simulink model "ROPOD_Control_SIM"  (R2017b)
settings: Solver=VariableStepAuto  StartTime=0.0  StopTime=inf  RelTol=1e-3
values from neighbouring files (symbols this model uses):
  AgentNumber = 1    [init_model.m]
  FFtheta_intia = 0    [init_model.m]
  FFxy_mass = 0*80    (= 0)    [init_model.m]
  flock_FFtheta_friction = 50    [init_model.m]
  flock_FFxy_friction = 100    [init_model.m]
  I_fhz_ddelta_cntr = 0    [init_model.m]
  I_fhz_dtheta_cntr = 0.3    [init_model.m]
  I_fhz_dtheta_flock_cntr = 0.1    [init_model.m]
  I_fhz_dvarphi_cntr = 0    [init_model.m]
  I_fhz_dxdy_cntr = 0.25    [init_model.m]
  I_fhz_dxdy_flock_cntr = 0.1    [init_model.m]
  K_gain_ddelta_cntr = 0.1    [init_model.m]
  K_gain_dtheta_cntr = 150    [init_model.m]
  K_gain_dtheta_flock_cntr = 100    [init_model.m]
  K_gain_dvarphi_cntr = 0.05    [init_model.m]
  K_gain_dxdy_cntr = 200    [init_model.m]
  K_gain_dxdy_flock_cntr = 200    [init_model.m]
  LL_wp_fhz_ddelta_cntr = 2    [init_model.m]
  LL_wp_fhz_dtheta_cntr = 20    [init_model.m]
  LL_wp_fhz_dtheta_flock_cntr = 20    [init_model.m]
  LL_wp_fhz_dvarphi_cntr = 10    [init_model.m]
  LL_wp_fhz_dxdy_cntr = 20    [init_model.m]
  LL_wp_fhz_dxdy_flock_cntr = 20    [init_model.m]
  LL_wz_fhz_ddelta_cntr = 2    [init_model.m]
  LL_wz_fhz_dtheta_cntr = 20    [init_model.m]
  LL_wz_fhz_dtheta_flock_cntr = 20    [init_model.m]
  LL_wz_fhz_dvarphi_cntr = 2    [init_model.m]
  LL_wz_fhz_dxdy_cntr = 20    [init_model.m]
  LL_wz_fhz_dxdy_flock_cntr = 20    [init_model.m]
  LPF_fhz_ddelta_cntr = 50    [init_model.m]
  LPF_fhz_ddelta_meas = 50    [init_model.m]
  LPF_fhz_dtheta_cntr = 100    [init_model.m]
  LPF_fhz_dtheta_flock_cntr = 40    [init_model.m]
  LPF_fhz_dvarphi_cntr = 50    [init_model.m]
  LPF_fhz_dvarphi_meas = 50    [init_model.m]
  LPF_fhz_dxdy_cntr = 100    [init_model.m]
  LPF_fhz_dxdy_flock_cntr = 40    [init_model.m]
  max_flock_acc_theta = 0.5    [init_model.m]
  max_flock_acc_xy = 0.5    [init_model.m]
  max_flock_vel_theta = 1.0    (= 1)    [init_model.m]
  max_flock_vel_xy = 1.0    (= 1)    [init_model.m]
  max_hw_tau = 7.0    (= 7)    [init_model.m]
  max_ropod_acc_theta = 1.6    [init_model.m]
  max_ropod_acc_xy = 2.0    (= 2)    [init_model.m]
  max_ropod_sw_force = 500    [init_model.m]
  max_ropod_sw_tau = 250    [init_model.m]
  max_ropod_vel_theta = 1.6    [init_model.m]
  max_ropod_vel_xy = 2.0    (= 2)    [init_model.m]
  max_sw_current = 10    [init_model.m]
  Nagents = 2    [init_model.m]
  Nwheels = 4    [Jqwl_numeric_function.m]    (also in S_matrix.m; extract_kinmodel_parameters.m; init_model.m; tau_optimal_dist_vec_fun.m)
  pivot_offs_sws = [0.0243    0.4689    0.3384    5.9050]    [init_model.m]
  ropod_kinmodel_pv = struct2array(ropod_kinmodel_param)    [set_ropod_KinModparams.m]
  ropod_position_inflock = [-1 0 3.1416]    [init_model.m]
  SW_COM1_ENABLE1 = hex2dec('0001')    [init_model.m]
  SW_COM1_ENABLE2 = hex2dec('0002')    [init_model.m]
  SW_COM1_MODE_TORQUE = bitshift(hex2dec('0000'),2)    [init_model.m]
  SW_COM1_MODE_VELOCITY = bitshift(hex2dec('0002'),2)    [init_model.m]
  SW_COM1_USE_TS = hex2dec('8000')    [init_model.m]
  sw_tau_2_current = 1/motor_physical_parameters.torqueconstant.value    [init_model.m]
  Tinit = 2    [init_model.m]
  Ts = 0.001    [init_model.m]
  Ts_MPC = 0.01    [init_model.m]
  Tsflck = 0.01    [init_model.m]
undefined symbols (not defined in the file or in its folder): acc_limit, accmax, b_cx, b_cy, b_rx, bus_size, comp_enable, Desired, DiscIntNeverNeededParam, Fcgain, gdis, k_cx, k_cy, live_tuning, m_robot, Nominal, Nominal_x, Nominal_y, offsets, portwidth, sizes, types, vel_limit, vmax1, vmax2
libraries: simulink x90, cstblocks x66, dspsigops x12, dspnetwork x4
(part 1 of 8)
settings Model: Creator=cesar  LastModifiedBy=cesar
settings OptimizationCC: DefaultParameterBehavior=Inlined  UseFloatMulNetSlope=on  InlineInvariantSignals=on  EfficientFloat2IntCast=on
settings DebuggingCC: UnderSpecifiedDataTypeMsg=warning
settings HardwareCC: ProdBitPerLong=64  ProdHWDeviceType=Intel->x86-64 (Linux 64)
settings RTWCC: GenCodeOnly=on  BuildConfiguration=Faster Runs
settings GRTTargetCC: MatFileLogging=off  SupportNonFinite=off

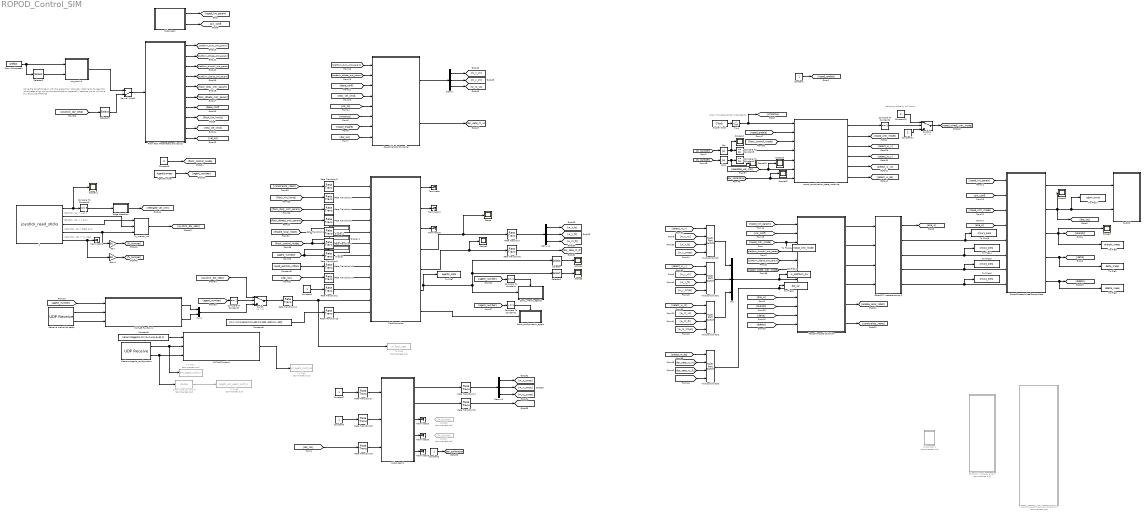
== system ROPOD_Control_SIM ==
  note: damping mode by full zmpc
  note: left stick - LR -> y axis
  note: Allow Tinit seconds for initialization
  note: doing the transformation with the angle from odometry data helps
      | to keep the robot better align during the Identification, especially because
      | we do not have any absolute reference
  note: left stick - UD -> x axis
  note: right stick - LR -> theta axis
  note: right stick - UD -> un used
  " 1" : S-Function  FunctionName=joystick_read_sticks  SFunctionDeploymentMode=off  EnableBusSupport=off  mask(Legacy Function){SFunctionSpec=double y1 = read_joystick(), ShowSpec=off}
      mask prompts: ShowSpec "Display function specification"
      mask help:
      | This block allows you to call the legacy functions specified by the following Legacy Code Tool definition:
      | def.SFunctionName = 'joystick_read';
      | def.OutputFcnSpec = 'double y1 = read_joystick()';
      | def.StartFcnSpec = 'void init()';
      | def.HeaderFiles = {'joystick.h', 'stdio.h', 'ncurses.h', 'gamepad.h'};
      | def.SourceFiles = {'joystick.c'};
      | def.HostLibFiles = {'libgamepad.so.1'};
      mask Help: <p>This block was generated automatically by the Legacy Code Tool. For detailed help on this tool, call<a href="matlab:legacy_code('help')"> legacy_code('help')</a>.</p>
      mask Callback ShowSpec:
      | if strcmp(get_param(gcbh, 'ShowSpec'), 'on')
      |   set_param(gcbh, 'MaskDisplay', sprintf('fprintf(''%s'');', get_param(gcbh, 'SFunctionSpec')));
      | else
      |   set_param(gcbh, 'MaskDisplay', sprintf('fprintf(''%s'');', get_param(gcbh, 'FunctionName')));
      | end
      mask Display: fprintf('joystick_read_sticks');
  Abs : Abs
  Abs1 : Abs
  AgentNumber : Constant  Value=AgentNumber
  Compare To Constant : simulink/Logic and Bit Operations/Compare To Constant  relop===  const=1  OutDataTypeStr=boolean
  Compare To Constant1 : simulink/Logic and Bit Operations/Compare To Constant  relop=~=  const=1  OutDataTypeStr=boolean
  Compare To Constant2 : simulink/Logic and Bit Operations/Compare To Constant  relop===  const=1  OutDataTypeStr=boolean
  Compare To Constant3 : simulink/Logic and Bit Operations/Compare To Constant  relop=>=  const=20  OutDataTypeStr=boolean
  Compare To Constant4 : simulink/Logic and Bit Operations/Compare To Constant  relop=>=  const=10  OutDataTypeStr=boolean
  Compare To Constant5 : simulink/Logic and Bit Operations/Compare To Constant  relop===  const=8  OutDataTypeStr=boolean
  Compare To Constant6 : simulink/Logic and Bit Operations/Compare To Constant  relop===  const=3  OutDataTypeStr=boolean
  Constant{,1..2,4,7} (5 alike) : Constant
  Constant10 : Constant  Value=3
  Constant11 : Constant  Value=2
  Constant5 : Constant  Value=0
  Constant6 : Constant  Value=[0 1 -1 0 3.1416 0 0 0 400 0 0 400 -400 0 0 -400]
  Constant8 : Constant  Value=zeros((Nagents-1)*(1+1+3+3+8),1)
  Constant9 : Constant  Value=ropod_position_inflock
  Data Type Conversion : DataTypeConversion  Commented=on  OutDataTypeStr=double
  Demux : Demux  Outputs=3
  Demux1 : Demux  Outputs=3
  Demux2 : Demux  Outputs=3
  Digital Clock : DigitalClock  SampleTime=Ts
  Display : Display
  Display1 : Display
  Display2 : Display
  Edge detection : Subsystem
  EtherCAT Interface empty : Subsystem  Commented=on
  EtherCAT Interface empty1 : Subsystem
  FlockController : Subsystem
  From Workspace1 : FromWorkspace  VariableName=qrefdot  SampleTime=Ts
  From ROS (Parameters and topics) : Subsystem
  Gain : Gain  Gain=50
  Gain1 : Gain  Gain=50
  Goto36 : Goto  Commented=on  GotoTag=fx_bumper
  Goto37 : Goto  Commented=on  GotoTag=fy_bumper
  MATLAB Function : MATLAB Function  TreatAsAtomicUnit=on
  MATLAB Function1 : MATLAB Function  TreatAsAtomicUnit=on
  Manual Switch : ManualSwitch  CurrentSetting=0
  Multiport Switch{,1..3} (4 alike) : MultiPortSwitch  DiagnosticForDefault=Warning
  Mux : Mux  Inputs=3
  Mux4 : Mux  Inputs=2
  Rate Transition{,6,14..15} (4 alike) : RateTransition  OutPortSampleTime=Ts
  Rate Transition{1..5,7..13} (12 alike) : RateTransition  OutPortSampleTime=Tsflck
  Rate Transition16 : RateTransition  OutPortSampleTime=Ts_MPC
  Rate Transition17 : RateTransition  OutPortSampleTime=Ts_MPC
  Rate Transition18 : RateTransition  OutPortSampleTime=Ts_MPC
  Recieve agents_configuration : dspnetwork/UDP Receive  localURL='0.0.0.0'  localPort=25002  remoteURL='0.0.0.0'  remotePort=-1  recvBufferSize=8192  dims=(1+1+3+3+8)  signalDatatype=double  isVarSize=off  showBlockingTime=on  blockingTime=0  sampletime=Ts  blockPlatform=HOST
      settings: SourceProductName=DSP System Toolbox  SourceProductBaseCode=DS
  Recieve wrench/dq setps : dspnetwork/UDP Receive  localURL='0.0.0.0'  localPort=25001  remoteURL='0.0.0.0'  remotePort=-1  recvBufferSize=8192  dims=2*3*(Nagents-1)  signalDatatype=double  isVarSize=off  showBlockingTime=on  blockingTime=0  sampletime=Ts  blockPlatform=HOST
      settings: SourceProductName=DSP System Toolbox  SourceProductBaseCode=DS
  RopodProcessWheelSensorData : Subsystem
  RopodProcessWheelSensorData_SIM : Subsystem  Commented=on
  RopodTorqueDistribution : Subsystem
  RopodVelocityController : Subsystem
  Scope{,1,3..6,11..15} (11 alike) : Scope
  Selector : Selector  InputPortWidth=6  IndexOptions=Index vector (dialog)  Indices=1:3  OutputSizes=1
  Selector1 : Selector  InputPortWidth=6  IndexOptions=Index vector (dialog)  Indices=4:6  OutputSizes=1
  Selector2 : Selector  InputPortWidth=3  IndexOptions=Index vector (dialog)  Indices=3  OutputSizes=1
  Selector3 : Selector  InputPortWidth=6  IndexOptions=Index vector (dialog)  Indices=[4:6]  OutputSizes=1
  Send_configuration_agent : Subsystem
  Send_wrench_agents : Subsystem
  Subsystem : Subsystem
  Subsystem1 : Subsystem  Commented=on
  Subsystem2 : Subsystem
  Switch : Switch  Criteria=u2 > Threshold
  Switch1 : Switch  Criteria=u2 > Threshold
  Terminator{,1..6} (7 alike) : Terminator
  "Tinit " : simulink/Logic and Bit Operations/Compare To Constant  relop=<  const=Tinit  OutDataTypeStr=boolean
  To File1 : ToFile  Filename=delta_meas  MatrixName=delta_meas
  To File10 : ToFile  Filename=dqr_sp  MatrixName=dqr_sp
  To File11 : ToFile  Filename=w_platform_sp  MatrixName=w_platform_sp
  To File12 : ToFile  Filename=ropod_cntr_mode  MatrixName=ropod_cntr_mode
  To File13 : ToFile  Filename=smw1_sens  MatrixName=smw1_sens  SampleTime=Ts
  To File14 : ToFile  Filename=smw2_sens  MatrixName=smw2_sens  SampleTime=Ts
  To File15 : ToFile  Filename=smw3_sens  MatrixName=smw3_sens  SampleTime=Ts
  To File16 : ToFile  Filename=smw4_sens  MatrixName=smw4_sens  SampleTime=Ts
  To File17 : ToFile  Filename=odom_twist  MatrixName=odom_twist
  To File3 : ToFile  Filename=ddelta_meas  MatrixName=ddelta_meas
  To File4 : ToFile  Commented=on  Filename=ext_agent_conf_in  MatrixName=ext_agent_conf_in
  To File5 : ToFile  Commented=on  Filename=length_ext_agent_conf_in  MatrixName=length_ext_agent_conf_in
  To File6 : ToFile  Commented=on  Filename=ext_agent_conf_out  MatrixName=ext_agent_conf_out
  To File7 : ToFile  Filename=agents_setp  MatrixName=agents_setp
  To File8 : ToFile  Commented=on  Filename=w_flock_setp  MatrixName=w_flock_setp
  To File9 : ToFile  Filename=dvarphi_meas  MatrixName=dvarphi_meas
  To_wrench_vel : Subsystem
  ropod_coordination_state_machine : MATLAB Function  TreatAsAtomicUnit=on
  rot_matrix2 : MATLAB Function  TreatAsAtomicUnit=on
  to_ROS : Subsystem
  wires:
  Rate Transition7/1 -> FlockController/5(enable_local_robot)
  EtherCAT Interface empty1/2(SW1_sens) -> To File13/1, RopodProcessWheelSensorData/5(SW1_sens)
  Multiport Switch3/1 -> To File10/1, RopodTorqueDistribution/8(dqr_sp_dvarphi_cntr)
  Compare To Constant/1 -> Send_wrench_agents/Enable
  [dvarphi] -> RopodTorqueDistribution/10(dvarphi)
  Constant5/1 -> [flock_control_mode]
  [dqr_loc] -> RopodVelocityController/8(dqr_loc)
  Recieve agents_configuration/1 -> To File4/1, MATLAB Function/2(message_in)
  [dqr_loc] -> Rate Transition11/1
  Constant8/1 -> MATLAB Function/1(ext_agents_configuration_ini)
  From ROS (Parameters and topics)/3(platform_dvarphi_cntr_param) -> [platform_dvarphi_cntr_param]
  [sw_conf] -> RopodProcessWheelSensorData/2(sw_conf)
  Compare To Constant2/1 -> Switch/2
  From ROS (Parameters and topics)/1(platform_dxdy_cntr_param) -> [platform_dxdy_cntr_param]
  Rate Transition4/1 -> FlockController/3(flock_dxdy_cntr_param)
  Rate Transition1/1 -> FlockController/2(flock_kin_limits)
  MATLAB Function/1(out_ext_agents_configuration) -> To File6/1
  [sw_conf] -> RopodTorqueDistribution/2(sw_conf)
  Rate Transition3/1 -> FlockController/1(constraints_local_robot)
  [agent_number] -> Compare To Constant2/1
  [ropod_wheel_cntr_mode] -> RopodTorqueDistribution/6(ropod_wheel_cntr_mode)
  [agent_number] -> MATLAB Function1/1(AgentNumber)
  [agent_number] -> Display/1, Rate Transition9/1
  RopodProcessWheelSensorData/3(dvarphi) -> Scope6/1, To File9/1, [dvarphi]
  Compare To Constant1/1 -> Send_configuration_agent/Enable
  [platform_ddelta_cntr_param] -> RopodTorqueDistribution/5(platform_ddelta_cntr_param)
  [vel_sp] -> RopodVelocityController/5(vel_sp)
  Rate Transition11/1 -> FlockController/9(dqr_loc)
  Subsystem/2(sw_conf) -> [sw_conf]
  [ropod_cntr_mode] -> RopodProcessWheelSensorData/3(ropod_cntr_mode)
  Constant9/1 -> Rate Transition10/1
  Constant/1 -> [ropod_enable]
  [ropod_enable] -> RopodVelocityController/7(ropod_enable)
  EtherCAT Interface empty1/3(SW2_sens) -> To File14/1, RopodProcessWheelSensorData/6(SW2_sens)
  Rate Transition13/1 -> FlockController/12(ext_agents_configuration)
  [ropod_cntr_mode] -> To File12/1, RopodTorqueDistribution/3(ropod_cntr_mode)
  [ena_w] -> RopodTorqueDistribution/9(ena_w)
  RopodTorqueDistribution/4(SW4_cmd) -> EtherCAT Interface empty1/4(SW4_cmd)
  [delta] -> RopodTorqueDistribution/11(delta)
  From ROS (Parameters and topics)/5(flock_dxdy_cntr_param) -> [flock_dxdy_cntr_param]
  [flock_kin_limits] -> Rate Transition1/1
  From ROS (Parameters and topics)/9(new_vel_cmd) -> [new_vel_cmd]
  Rate Transition9/1 -> FlockController/7(agent_number)
  [agent_number] -> Compare To Constant1/1
  RopodTorqueDistribution/5(enable_robot) -> [enable_local_robot]
  RopodTorqueDistribution/2(SW2_cmd) -> EtherCAT Interface empty1/2(SW2_cmd)
  Rate Transition8/1 -> FlockController/6(flock_control_mode)
  RopodTorqueDistribution/3(SW3_cmd) -> EtherCAT Interface empty1/3(SW3_cmd)
  From ROS (Parameters and topics)/6(flock_dtheta_cntr_param) -> [flock_dtheta_cntr_param]
  RopodProcessWheelSensorData/2(odom_robot_twist) -> Scope3/1, [dqr_loc], To File17/1, to_ROS/2(odom_robot_twist)
  [flock_dtheta_cntr_param] -> Rate Transition5/1
  RopodTorqueDistribution/1(SW1_cmd) -> EtherCAT Interface empty1/1(SW1_cmd)
  [enable_local_robot] -> Display2/1, Rate Transition7/1
  [constraints_robot] -> Rate Transition3/1
  EtherCAT Interface empty1/4(SW3_sens) -> To File15/1, RopodProcessWheelSensorData/7(SW3_sens)
  [flock_dxdy_cntr_param] -> Rate Transition4/1
  EtherCAT Interface empty1/1(ena_w) -> [ena_w]
  [ropod_kin_param] -> RopodProcessWheelSensorData/1(ropod_kin_param)
  [ddelta] -> RopodTorqueDistribution/12(ddelta)
  RopodProcessWheelSensorData/1(odom_robot_pose) -> to_ROS/1(odom_robot_pose)
  [select_w_x] -> Multiport Switch/1
  Recieve agents_configuration/2 -> Data Type Conversion/1, MATLAB Function/3(length_in)
  [ropod_kin_param] -> RopodTorqueDistribution/1(ropod_kinmodel_pv)
  [agent_number] -> Compare To Constant/1
  Recieve wrench/dq setps/2 -> MATLAB Function1/3(length_msg)
  [base_conf] -> RopodVelocityController/3(base_conf)
  [platform_dvarphi_cntr_param] -> RopodTorqueDistribution/4(platform_dvarphi_cntr_param)
  Data Type Conversion/1 -> To File5/1
  [flock_control_mode] -> Display1/1, Rate Transition8/1
  FlockController/4(w_platform_setp) -> Scope/1, Rate Transition/1
  [new_vel_cmd] -> RopodVelocityController/4(new_vel_cmd)
  Mux/1 -> To File11/1, RopodTorqueDistribution/7(w_platform_setp)
  Rate Transition10/1 -> FlockController/8(position_inflock)
  From ROS (Parameters and topics)/2(platform_dtheta_cntr_param) -> [platform_dtheta_cntr_param]
  Recieve wrench/dq setps/1 -> MATLAB Function1/2(message_in)
  " 1"/5 -> Gain1/1, Terminator1/1
  Subsystem/1(ropod_kin_param) -> [ropod_kin_param]
  FlockController/7(local_agent_configuration) -> Send_configuration_agent/1(local_agent_configuration)
  AgentNumber/1 -> [agent_number]  "agent_number"
  From ROS (Parameters and topics)/4(platform_ddelta_cntr_param) -> [platform_ddelta_cntr_param]
  [initialize] -> RopodVelocityController/6(initialize)
  Switch/1 -> Rate Transition12/1
  [platform_dtheta_cntr_param] -> RopodVelocityController/2(platform_dtheta_cntr_param)
  From ROS (Parameters and topics)/7(base_conf) -> [base_conf]
  Rate Transition12/1 -> To File8/1, FlockController/11(flock_sp)
  RopodProcessWheelSensorData/5(ddelta) -> To File3/1, [ddelta]
  RopodTorqueDistribution/6(constraints_robot) -> [constraints_robot]
  " 1"/1 -> Scope11/1, Compare To Constant5/1
  [platform_dxdy_cntr_param] -> RopodVelocityController/1(platform_dxdy_cntr_param)
  FlockController/5(dq_platform_setp) -> Scope1/1, Rate Transition6/1
  RopodProcessWheelSensorData/4(delta) -> To File1/1, [delta]
  Rate Transition5/1 -> FlockController/4(flock_dtheta_cntr_param)
  From ROS (Parameters and topics)/8(flock_kin_limits) -> [flock_kin_limits]
  Constant1/1 -> Rate Transition2/1
  [ena_w] -> RopodProcessWheelSensorData/4(ena_w)
  Rate Transition2/1 -> FlockController/10(new_cmd)
  FlockController/6(agents_setp) -> To File7/1, Send_wrench_agents/1(w_dq_agents_setp), Selector1/1, Selector/1
  MATLAB Function1/1(WrenchAgent) -> Mux4/1
  MATLAB Function1/2(dqAgent) -> Mux4/2
  Mux4/1 -> Switch/3
  " 1"/2 -> To_wrench_vel/2(y)
  Constant6/1 -> Rate Transition13/1
  Selector/1 -> Scope4/1
  Selector1/1 -> Scope5/1
  FlockController/1(w_flock_setp) -> Terminator/1
  FlockController/2(dq_flock_setp) -> Terminator4/1
  FlockController/3(flock_aplha) -> Terminator5/1
  EtherCAT Interface empty1/5(SW4_sens) -> To File16/1, RopodProcessWheelSensorData/8(SW4_sens)
  [dqr_loc] -> Rate Transition16/1
  Rate Transition16/1 -> Subsystem2/3(dqr_loc)
  " 1"/4 -> Gain/1, To_wrench_vel/3(theta)
  Subsystem2/1(w_platform_setp) -> Rate Transition14/1
  Subsystem2/2(dq_platform_setp) -> Rate Transition15/1
  Constant4/1 -> Rate Transition18/1
  Constant7/1 -> Rate Transition17/1
  Rate Transition17/1 -> Subsystem2/1(zmpc_x_enable)
  Rate Transition18/1 -> Subsystem2/2(zmpc_y_enable)
  Demux/1 -> [w_x_vc]
  Demux/2 -> [w_y_vc]
  Demux/3 -> [w_rz_vc]
  RopodVelocityController/1(w_platform_setp) -> Demux/1
  RopodVelocityController/2(dqr_sp_dvarphi_cntr) -> [dqr_setp_rz_vc]
  [select_w_y] -> Multiport Switch1/1
  [select_w_rz] -> Multiport Switch2/1
  [select_w_dq] -> Multiport Switch3/1
  Multiport Switch1/1 -> Mux/2
  Multiport Switch/1 -> Mux/1
  Multiport Switch2/1 -> Mux/3
  Demux1/3 -> [w_rz_fc]
  Demux1/1 -> [w_x_fc]
  Rate Transition/1 -> Demux1/1
  Demux1/2 -> [w_y_fc]
  [w_x_vc] -> Multiport Switch/2
  [w_x_fc] -> Multiport Switch/3
  [w_y_vc] -> Multiport Switch1/2
  [w_rz_vc] -> Multiport Switch2/2
  [dqr_setp_rz_vc] -> Multiport Switch3/2
  [w_y_fc] -> Multiport Switch1/3
  [w_rz_fc] -> Multiport Switch2/3
  Rate Transition6/1 -> [dqr_setp_rz_fc]
  [dqr_setp_rz_fc] -> Multiport Switch3/3
  Demux2/1 -> [w_x_zmpc]
  Rate Transition14/1 -> Demux2/1
  Rate Transition15/1 -> [dqr_setp_rz_zmpc]
  Demux2/3 -> [w_rz_zmpc]
  Demux2/2 -> [w_y_zmpc]
  [w_x_zmpc] -> Multiport Switch/4
  [w_y_zmpc] -> Multiport Switch1/4
  [w_rz_zmpc] -> Multiport Switch2/4
  [dqr_setp_rz_zmpc] -> Multiport Switch3/4
  Digital Clock/1 -> "Tinit "/1
  [ropod_enable] -> ropod_coordination_state_machine/2(ropod_enable)
  ropod_coordination_state_machine/2(ropod_cntr_mode) -> [ropod_cntr_mode]
  "Tinit "/1 -> [initialize], ropod_coordination_state_machine/1(initialize)
  [fx_bumper] -> Abs/1
  Abs/1 -> Scope12/1, Compare To Constant3/1
  Abs1/1 -> Scope13/1, Compare To Constant4/1
  [fy_bumper] -> Abs1/1
  Compare To Constant3/1 -> ropod_coordination_state_machine/4(enable_zmpc_fx)
  Compare To Constant4/1 -> ropod_coordination_state_machine/5(enable_zmpc_fy)
  [reenable_vel_cntr] -> Scope14/1, ropod_coordination_state_machine/6(reenable_vel_cntr)
  [flock_control_mode] -> ropod_coordination_state_machine/3(flock_mode)
  ropod_coordination_state_machine/3(select_w_x) -> [select_w_x]
  ropod_coordination_state_machine/4(select_w_y) -> [select_w_y]
  ropod_coordination_state_machine/5(select_w_rz) -> [select_w_rz]
  ropod_coordination_state_machine/6(select_dq) -> [select_w_dq]
  To_wrench_vel/1(Out1) -> [joystick_dqr_setp]
  [joystick_dqr_setp] -> Switch/1
  From Workspace1/1 -> Selector2/1, rot_matrix2/1(dqr_glb)
  rot_matrix2/1(dqr_loc) -> Manual Switch/1
  Selector2/1 -> rot_matrix2/2(theta)
  [joystick_dqr_setp] -> Selector3/1
  Selector3/1 -> Manual Switch/2
  Manual Switch/1 -> From ROS (Parameters and topics)/1(vsep_in)
  From ROS (Parameters and topics)/10(vel_sp) -> [vel_sp]
  " 1"/3 -> To_wrench_vel/1(x)
  Subsystem2/3(Fx) -> Terminator2/1
  Subsystem2/4(Fy) -> Terminator3/1
  Subsystem2/5(bumper_cal_done) -> Terminator6/1
  Constant2/1 -> [bpr_calibration]
  Gain/1 -> [fy_bumper]
  Gain1/1 -> [fx_bumper]
  [bpr_calibration] -> Scope15/1, ropod_coordination_state_machine/7(bpr_calibration)
  Compare To Constant5/1 -> Edge detection/1(In1)
  Edge detection/1(Out1) -> [reenable_vel_cntr]
  ropod_coordination_state_machine/1(ropod_cntr_state) -> Compare To Constant6/1
  Switch1/1 -> [ropod_wheel_cntr_mode]
  Compare To Constant6/1 -> Switch1/2
  Constant10/1 -> Switch1/1
  Constant11/1 -> Switch1/3

== system ROPOD_Control_SIM/Edge detection ==
  In1 : Inport
  Compare To Zero : simulink/Logic and Bit Operations/Compare To Zero  relop===  OutDataTypeStr=boolean
  Compare To Zero1 : simulink/Logic and Bit Operations/Compare To Zero  relop=>  OutDataTypeStr=boolean
  Logical Operator : Logic  AllPortsSameDT=off  OutDataTypeStr=boolean
  Unit Delay : UnitDelay  SampleTime=-1
  Out1 : Outport
  wires:
  Compare To Zero1/1 -> Logical Operator/2
  In1/1 -> Unit Delay/1, Compare To Zero1/1
  Unit Delay/1 -> Compare To Zero/1
  Logical Operator/1 -> Out1/1
  Compare To Zero/1 -> Logical Operator/1

== system ROPOD_Control_SIM/EtherCAT Interface empty ==
  SW1_cmd : Inport
  SW2_cmd : Inport  Port=2
  SW3_cmd : Inport  Port=3
  SW4_cmd : Inport  Port=4
  Constant : Constant  Value=[1 0 1 0]
  empywheel : Subsystem
  empywheel1 : Subsystem
  empywheel2 : Subsystem
  empywheel3 : Subsystem
  ena_w : Outport
  SW1_sens : Outport  Port=2
  SW2_sens : Outport  Port=3
  SW3_sens : Outport  Port=4
  SW4_sens : Outport  Port=5
  wires:
  empywheel1/1(SW4_sens) -> SW2_sens/1  "SW2_sens"
  empywheel2/1(SW4_sens) -> SW3_sens/1  "SW3_sens"
  SW4_cmd/1 -> empywheel3/1(SW4_cmd)
  SW2_cmd/1 -> empywheel1/1(SW4_cmd)
  SW3_cmd/1 -> empywheel2/1(SW4_cmd)
  SW1_cmd/1 -> empywheel/1(SW4_cmd)
  empywheel/1(SW4_sens) -> SW1_sens/1  "SW1_sens"
  empywheel3/1(SW4_sens) -> SW4_sens/1  "SW4_sens"
  Constant/1 -> ena_w/1

== system ROPOD_Control_SIM/EtherCAT Interface empty1 ==
  SW1_cmd : Inport
  SW2_cmd : Inport  Port=2
  SW3_cmd : Inport  Port=3
  SW4_cmd : Inport  Port=4
  Constant : Constant  Value=[1 0 1 0]
  empywheel : Subsystem
  empywheel1 : Subsystem
  empywheel2 : Subsystem
  empywheel3 : Subsystem
  ena_w : Outport
  SW1_sens : Outport  Port=2
  SW2_sens : Outport  Port=3
  SW3_sens : Outport  Port=4
  SW4_sens : Outport  Port=5
  wires:
  empywheel1/1(SW4_sens) -> SW2_sens/1  "SW2_sens"
  empywheel2/1(SW4_sens) -> SW3_sens/1  "SW3_sens"
  SW4_cmd/1 -> empywheel3/1(SW4_cmd)
  SW2_cmd/1 -> empywheel1/1(SW4_cmd)
  SW3_cmd/1 -> empywheel2/1(SW4_cmd)
  SW1_cmd/1 -> empywheel/1(SW4_cmd)
  empywheel/1(SW4_sens) -> SW1_sens/1  "SW1_sens"
  empywheel3/1(SW4_sens) -> SW4_sens/1  "SW4_sens"
  Constant/1 -> ena_w/1

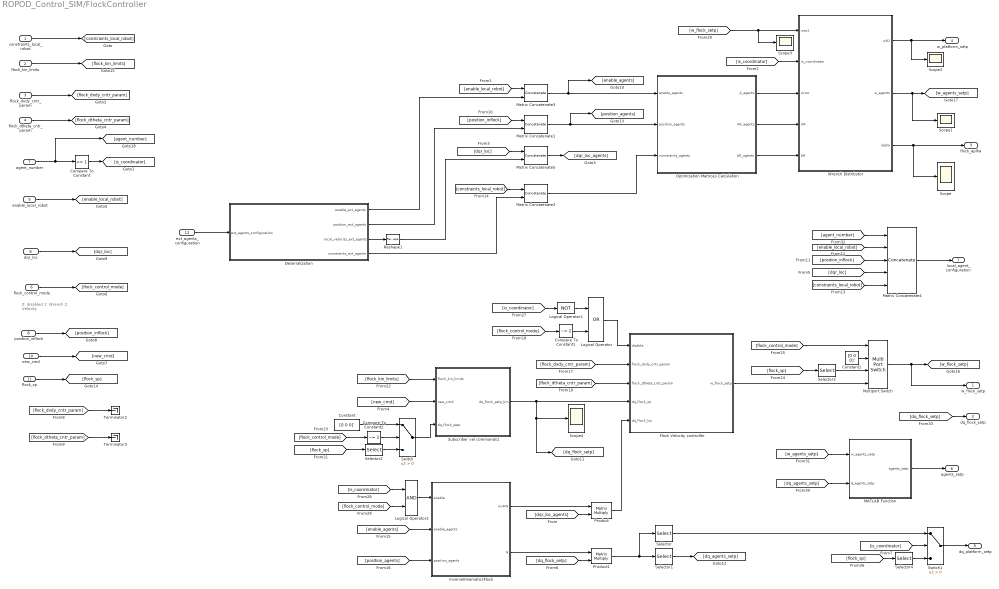
== system ROPOD_Control_SIM/FlockController ==
  note: 0: disabled
      | 1: Wrench
      | 2: Velocity
  constraints_local_robot : Inport
  flock_kin_limits : Inport  Port=2
  flock_dxdy_cntr_param : Inport  Port=3
  flock_dtheta_cntr_param : Inport  Port=4
  enable_local_robot : Inport  Port=5
  flock_control_mode : Inport  Port=6
  agent_number : Inport  Port=7
  position_inflock : Inport  Port=8
  dqr_loc : Inport  Port=9
  new_cmd : Inport  Port=10
  flock_sp : Inport  Port=11
  ext_agents_configuration : Inport  Port=12
  Compare To Constant : simulink/Logic and Bit Operations/Compare To Constant  relop===  const=1  OutDataTypeStr=boolean
  Compare To Constant1 : simulink/Logic and Bit Operations/Compare To Constant  relop=~=  const=2  OutDataTypeStr=boolean
  Compare To Constant2 : simulink/Logic and Bit Operations/Compare To Constant  relop=~=  const=2  OutDataTypeStr=boolean
  Constant : Constant  Value=[0 0 0]'
  Constant1 : Constant  Value=[0 0 0]'
  Deserialization : MATLAB Function  TreatAsAtomicUnit=on
  Flock Velocity controller : Subsystem
  InverseKinematicsFlock : MATLAB Function  TreatAsAtomicUnit=on
  Logical Operator : Logic  Operator=OR  AllPortsSameDT=off  OutDataTypeStr=boolean
  Logical Operator1 : Logic  Operator=NOT  AllPortsSameDT=off  OutDataTypeStr=boolean
  Logical Operator2 : Logic  AllPortsSameDT=off  OutDataTypeStr=boolean
  MATLAB Function : MATLAB Function  TreatAsAtomicUnit=on
  Matrix Concatenate1 : Concatenate  Mode=Multidimensional array  ConcatenateDimension=2
  Matrix Concatenate2 : Concatenate  Mode=Multidimensional array  ConcatenateDimension=2
  Matrix Concatenate3 : Concatenate  Mode=Multidimensional array  ConcatenateDimension=2
  Matrix Concatenate4 : Concatenate  NumInputs=5  Mode=Multidimensional array
  Matrix Concatenate5 : Concatenate  Mode=Multidimensional array
  Multiport Switch : MultiPortSwitch  DataPortOrder=Zero-based contiguous
  Optimization Matrices Calculation : MATLAB Function  TreatAsAtomicUnit=on
  Product : Product  Multiplication=Matrix(*)
  Product1 : Product  Multiplication=Matrix(*)
  Reshape1 : Reshape
  Scope{,1..4} (5 alike) : Scope
  Selector : Selector  InputPortWidth=3*Nagents  IndexOptions=Index vector (dialog)  Indices=1:3  OutputSizes=1
  Selector1 : Selector  InputPortWidth=3*Nagents  IndexOptions=Index vector (dialog)  Indices=4:Nagents*3  OutputSizes=1
  Selector2 : Selector  InputPortWidth=6  IndexOptions=Index vector (dialog)  Indices=4:6  OutputSizes=1
  Selector3 : Selector  InputPortWidth=6  IndexOptions=Index vector (dialog)  Indices=1:3  OutputSizes=1
  Selector4 : Selector  InputPortWidth=6  IndexOptions=Index vector (dialog)  Indices=4:6  OutputSizes=1
  Subscriber vel commands1 : Subsystem
  Switch : Switch  Criteria=u2 > Threshold
  Switch1 : Switch  Criteria=u2 > Threshold
  Terminator2 : Terminator
  Terminator3 : Terminator
  Wrench Distributor : MATLAB Function  TreatAsAtomicUnit=on
  w_flock_setp : Outport
  dq_flock_setp : Outport  Port=2
  flock_aplha : Outport  Port=3
  w_platform_setp : Outport  Port=4
  dq_platform_setp : Outport  Port=5
  agents_setp : Outport  Port=6
  local_agent_configuration : Outport  Port=7
  wires:
  constraints_local_robot/1 -> [constraints_local_robot]
  Wrench Distributor/1(wR1) -> Scope2/1, w_platform_setp/1
  agent_number/1 -> [agent_number], Compare To Constant/1
  [is_coordinator] -> Wrench Distributor/2(is_coordinator)
  Wrench Distributor/2(w_agents) -> [w_agents_setp], Scope1/1
  Wrench Distributor/3(alpha) -> flock_aplha/1, Scope/1
  flock_dxdy_cntr_param/1 -> [flock_dxdy_cntr_param]
  flock_dtheta_cntr_param/1 -> [flock_dtheta_cntr_param]
  ext_agents_configuration/1 -> Deserialization/1(ext_agents_configuration)
  Optimization Matrices Calculation/1(A_agents) -> Wrench Distributor/3(Arow)
  Optimization Matrices Calculation/2(AR_agents) -> Wrench Distributor/4(AR)
  Optimization Matrices Calculation/3(bR_agents) -> Wrench Distributor/5(bR)
  Matrix Concatenate2/1 -> Optimization Matrices Calculation/3(constraints_agents)
  Matrix Concatenate1/1 -> [position_agents], Optimization Matrices Calculation/2(position_agents)
  Matrix Concatenate3/1 -> [enable_agents], Optimization Matrices Calculation/1(enable_agents)
  dqr_loc/1 -> [dqr_loc]
  enable_local_robot/1 -> [enable_local_robot]
  [enable_local_robot] -> Matrix Concatenate3/1
  flock_control_mode/1 -> [flock_control_mode]
  [flock_dxdy_cntr_param] -> Terminator2/1
  [flock_dtheta_cntr_param] -> Terminator3/1
  Matrix Concatenate4/1 -> local_agent_configuration/1
  position_inflock/1 -> [position_inflock]
  [position_inflock] -> Matrix Concatenate1/1
  Compare To Constant/1 -> [is_coordinator]
  [dqr_loc] -> Matrix Concatenate5/1
  [constraints_local_robot] -> Matrix Concatenate2/1
  [position_agents] -> InverseKinematicsFlock/3(position_agents)
  [enable_agents] -> InverseKinematicsFlock/2(enable_agents)
  [flock_dxdy_cntr_param] -> Flock Velocity controller/2(flock_dxdy_cntr_param)
  [flock_dtheta_cntr_param] -> Flock Velocity controller/3(flock_dtheta_cntr_param)
  [flock_control_mode] -> Compare To Constant1/1
  [w_flock_setp] -> Scope3/1, Wrench Distributor/1(wact)
  flock_sp/1 -> [flock_sp]
  flock_kin_limits/1 -> [flock_kin_limits]
  [flock_kin_limits] -> Subscriber vel commands1/1(flock_kin_limits)
  Subscriber vel commands1/1(dq_flock_setp_lim) -> Flock Velocity controller/4(dq_flock_sp), [dq_flock_setp], Scope4/1
  Compare To Constant2/1 -> Switch/2
  [flock_sp] -> Selector2/1
  [flock_control_mode] -> Compare To Constant2/1
  Constant/1 -> Switch/1
  [flock_control_mode] -> Multiport Switch/1
  Constant1/1 -> Multiport Switch/2
  Flock Velocity controller/1(w_flock_setp) -> Multiport Switch/4
  Switch/1 -> Subscriber vel commands1/3(dq_flock_setp)
  new_cmd/1 -> [new_cmd]
  [new_cmd] -> Subscriber vel commands1/2(new_cmd)
  Deserialization/3(local_velocity_ext_agents) -> Reshape1/1
  Matrix Concatenate5/1 -> [dqr_loc_agents]
  InverseKinematicsFlock/1(invMG) -> Product/1
  [dqr_loc_agents] -> Product/2
  Product/1 -> Flock Velocity controller/5(dq_flock_loc)
  InverseKinematicsFlock/2(G) -> Product1/1
  [dq_flock_setp] -> Product1/2
  Product1/1 -> Selector/1, Selector1/1
  Selector2/1 -> Switch/3
  [flock_sp] -> Selector3/1
  Selector3/1 -> Multiport Switch/3
  Switch1/1 -> dq_platform_setp/1
  [is_coordinator] -> Switch1/2
  Selector/1 -> Switch1/1
  [flock_sp] -> Selector4/1
  Selector4/1 -> Switch1/3
  Compare To Constant1/1 -> Logical Operator/2
  [is_coordinator] -> Logical Operator1/1
  Logical Operator1/1 -> Logical Operator/1
  Logical Operator/1 -> Flock Velocity controller/1(disable)
  [is_coordinator] -> Logical Operator2/1
  [flock_control_mode] -> Logical Operator2/2
  Logical Operator2/1 -> InverseKinematicsFlock/1(enable)
  Multiport Switch/1 -> w_flock_setp/1, [w_flock_setp]
  Selector1/1 -> [dq_agents_setp]
  [dq_agents_setp] -> MATLAB Function/2(d_agents_setp)
  MATLAB Function/1(agents_setp) -> agents_setp/1
  [w_agents_setp] -> MATLAB Function/1(w_agents_setp)
  Deserialization/4(constraints_ext_agents) -> Matrix Concatenate2/2
  Reshape1/1 -> Matrix Concatenate5/2
  Deserialization/2(position_ext_agents) -> Matrix Concatenate1/2
  Deserialization/1(enable_ext_agents) -> Matrix Concatenate3/2
  [agent_number] -> Matrix Concatenate4/1
  [enable_local_robot] -> Matrix Concatenate4/2
  [position_inflock] -> Matrix Concatenate4/3
  [dqr_loc] -> Matrix Concatenate4/4
  [constraints_local_robot] -> Matrix Concatenate4/5
  [dq_flock_setp] -> dq_flock_setp/1

== system ROPOD_Control_SIM/From ROS (Parameters and topics) ==
  vsep_in : Inport
  Constant1 : Constant
  Controllers conf : Subsystem
  Gain1 : Gain
  ROS base conf : Subsystem
  flock kin limits : Subsystem
  platform_dxdy_cntr_param : Outport
  platform_dtheta_cntr_param : Outport  Port=2
  platform_dvarphi_cntr_param : Outport  Port=3
  platform_ddelta_cntr_param : Outport  Port=4
  flock_dxdy_cntr_param : Outport  Port=5
  flock_dtheta_cntr_param : Outport  Port=6
  base_conf : Outport  Port=7
  flock_kin_limits : Outport  Port=8
  new_vel_cmd : Outport  Port=9
  vel_sp : Outport  Port=10
  wires:
  Controllers conf/1(platform_dxdy_cntr_param) -> platform_dxdy_cntr_param/1
  Constant1/1 -> new_vel_cmd/1
  Gain1/1 -> vel_sp/1
  ROS base conf/1(base_conf) -> base_conf/1
  Controllers conf/3(platform_dvarphi_cntr_param) -> platform_dvarphi_cntr_param/1
  Controllers conf/2(platform_dtheta_cntr_param) -> platform_dtheta_cntr_param/1
  Controllers conf/4(platform_ddelta_cntr_param) -> platform_ddelta_cntr_param/1
  Controllers conf/5(flock_dxdy_cntr_param) -> flock_dxdy_cntr_param/1
  Controllers conf/6(flock_dtheta_cntr_param) -> flock_dtheta_cntr_param/1
  flock kin limits/1(flock_kin_limits) -> flock_kin_limits/1
  vsep_in/1 -> Gain1/1

== system ROPOD_Control_SIM/RopodProcessWheelSensorData ==
  ropod_kin_param : Inport
  sw_conf : Inport  Port=2
  ropod_cntr_mode : Inport  Port=3
  ena_w : Inport  Port=4
  SW1_sens : Inport  Port=5
  SW2_sens : Inport  Port=6
  SW3_sens : Inport  Port=7
  SW4_sens : Inport  Port=8
  Compare To Constant : simulink/Logic and Bit Operations/Compare To Constant  relop=~=  const=1  OutDataTypeStr=boolean
  Odometry and Measurement model 4SW : Subsystem
  ROPOD_4Wheel_sens : Subsystem
  odom_robot_pose : Outport
  odom_robot_twist : Outport  Port=2
  dvarphi : Outport  Port=3
  delta : Outport  Port=4
  ddelta : Outport  Port=5
  wires:
  ropod_kin_param/1 -> Odometry and Measurement model 4SW/1(param_in)
  Odometry and Measurement model 4SW/2(odom_robot_twist) -> odom_robot_twist/1
  SW2_sens/1 -> ROPOD_4Wheel_sens/4(SW2_sens)
  ROPOD_4Wheel_sens/3(ddelta) -> ddelta/1
  Odometry and Measurement model 4SW/1(odom_robot_pose) -> odom_robot_pose/1
  ROPOD_4Wheel_sens/2(delta) -> Odometry and Measurement model 4SW/4(delta), delta/1
  SW4_sens/1 -> ROPOD_4Wheel_sens/6(SW4_sens)
  ROPOD_4Wheel_sens/1(dvarphi) -> Odometry and Measurement model 4SW/3(dvarphi), dvarphi/1
  SW3_sens/1 -> ROPOD_4Wheel_sens/5(SW3_sens)
  SW1_sens/1 -> ROPOD_4Wheel_sens/3(SW1_sens)
  Compare To Constant/1 -> ROPOD_4Wheel_sens/1(disable)
  sw_conf/1 -> ROPOD_4Wheel_sens/2(sw_conf)
  ropod_cntr_mode/1 -> Compare To Constant/1
  ena_w/1 -> Odometry and Measurement model 4SW/2(ena_w)

== system ROPOD_Control_SIM/RopodProcessWheelSensorData_SIM ==
  ropod_kin_param : Inport
  sw_conf : Inport  Port=2
  ropod_cntr_mode : Inport  Port=3
  ena_w : Inport  Port=4
  SW1_sens : Inport  Port=5
  SW2_sens : Inport  Port=6
  SW3_sens : Inport  Port=7
  SW4_sens : Inport  Port=8
  Compare To Constant : simulink/Logic and Bit Operations/Compare To Constant  relop=~=  const=1  OutDataTypeStr=boolean
  Odometry and Measurement model 4SW : Subsystem
  ROPOD_4Wheel_sens : Subsystem
  odom_robot_pose : Outport
  odom_robot_twist : Outport  Port=2
  dvarphi : Outport  Port=3
  delta : Outport  Port=4
  ddelta : Outport  Port=5
  wires:
  ropod_kin_param/1 -> Odometry and Measurement model 4SW/1(param_in)
  Odometry and Measurement model 4SW/2(odom_robot_twist) -> odom_robot_twist/1
  SW2_sens/1 -> ROPOD_4Wheel_sens/4(SW2_sens)
  ROPOD_4Wheel_sens/3(ddelta) -> ddelta/1
  Odometry and Measurement model 4SW/1(odom_robot_pose) -> odom_robot_pose/1
  ROPOD_4Wheel_sens/2(delta) -> Odometry and Measurement model 4SW/4(delta), delta/1
  SW4_sens/1 -> ROPOD_4Wheel_sens/6(SW4_sens)
  ROPOD_4Wheel_sens/1(dvarphi) -> Odometry and Measurement model 4SW/3(dvarphi), dvarphi/1
  SW3_sens/1 -> ROPOD_4Wheel_sens/5(SW3_sens)
  SW1_sens/1 -> ROPOD_4Wheel_sens/3(SW1_sens)
  Compare To Constant/1 -> ROPOD_4Wheel_sens/1(disable)
  sw_conf/1 -> ROPOD_4Wheel_sens/2(sw_conf)
  ropod_cntr_mode/1 -> Compare To Constant/1
  ena_w/1 -> Odometry and Measurement model 4SW/2(ena_w)

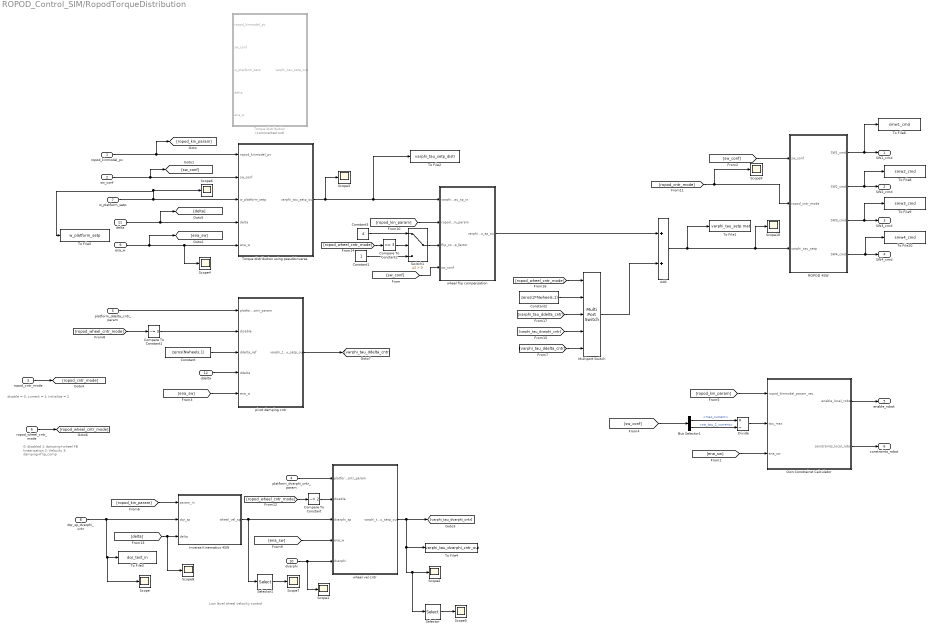
== system ROPOD_Control_SIM/RopodTorqueDistribution ==
  note: Low level wheel velocity control
  note: 0: disabled
      | 1: damping+wheel FB linearization
      | 2: Velocity
      | 3: damping+flip_comp
  note: disable = 0, current = 1, initialize = 2
  ropod_kinmodel_pv : Inport
  sw_conf : Inport  Port=2
  ropod_cntr_mode : Inport  Port=3
  platform_dvarphi_cntr_param : Inport  Port=4
  platform_ddelta_cntr_param : Inport  Port=5
  ropod_wheel_cntr_mode : Inport  Port=6
  w_platform_setp : Inport  Port=7
  dqr_sp_dvarphi_cntr : Inport  Port=8
  ena_w : Inport  Port=9
  dvarphi : Inport  Port=10
  delta : Inport  Port=11
  ddelta : Inport  Port=12
  Add : Sum
  Bus Selector1 : BusSelector  OutputSignals=max_current,sw_tau_2_current
  Compare To Constant : simulink/Logic and Bit Operations/Compare To Constant  relop=~=  const=2  OutDataTypeStr=boolean
  Compare To Constant1 : simulink/Logic and Bit Operations/Compare To Constant  relop=~=  const=3  OutDataTypeStr=boolean
  Compare To Constant2 : simulink/Logic and Bit Operations/Compare To Constant  relop===  const=3  OutDataTypeStr=boolean
  Constant : Constant  Value=zeros(Nwheels,1)
  Constant1 : Constant
  Constant2 : Constant  Value=zeros(2*Nwheels,1)
  Constant3 : Constant  Value=4
  Divide : Product  Inputs=*/
  Inverse Kinematics 4SW : Subsystem
  Multiport Switch : MultiPortSwitch  DataPortOrder=Zero-based contiguous  Inputs=4
  Own Constrainst Calculator : MATLAB Function  TreatAsAtomicUnit=on
  ROPOD 4SW : Subsystem
  Scope{,1..10} (11 alike) : Scope
  Selector : Selector  InputPortWidth=8  IndexOptions=Index vector (dialog)  Indices=1  OutputSizes=1
  Selector1 : Selector  InputPortWidth=8  IndexOptions=Index vector (dialog)  Indices=1  OutputSizes=1
  Switch1 : Switch  Criteria=u2 > Threshold
  To File1 : ToFile  Filename=varphi_tau_setp.mat  MatrixName=varphi_tau_setp
  To File10 : ToFile  Filename=smw4_cmd  MatrixName=smw4_cmd
  To File2 : ToFile  Filename=varphi_tau_setp_distr  MatrixName=varphi_tau_setp_distr
  To File3 : ToFile  Filename=dqr_test_in  MatrixName=dqr_test_in
  To File4 : ToFile  Filename=varphi_tau_dvarphi_cntr_out  MatrixName=varphi_tau_dvarphi_cntr_out
  To File5 : ToFile  Filename=w_platform_setp  MatrixName=w_platform_setp
  To File6 : ToFile  Filename=smw1_cmd  MatrixName=smw1_cmd
  To File8 : ToFile  Filename=smw2_cmd  MatrixName=smw2_cmd
  To File9 : ToFile  Filename=smw3_cmd  MatrixName=smw3_cmd
  Torque distribution : Subsystem  Commented=on
  Torque distribution using pseudoinverse : Subsystem
  pivot damping cntr : Subsystem
  wheel flip compensation : Subsystem
  wheel vel cntr : Subsystem
  SW1_cmd : Outport
  SW2_cmd : Outport  Port=2
  SW3_cmd : Outport  Port=3
  SW4_cmd : Outport  Port=4
  enable_robot : Outport  Port=5
  constraints_robot : Outport  Port=6
  wires:
  ROPOD 4SW/4(SW4_cmd) -> To File10/1, SW4_cmd/1
  w_platform_setp/1 -> Torque distribution using pseudoinverse/3(w_platform_setp), To File5/1, Scope6/1
  ropod_kinmodel_pv/1 -> Torque distribution using pseudoinverse/1(ropod_kinmodel_pv), [ropod_kin_param]
  ROPOD 4SW/1(SW1_cmd) -> To File6/1, SW1_cmd/1
  ena_w/1 -> Torque distribution using pseudoinverse/5(ena_w), Scope4/1, [ena_sw]
  ROPOD 4SW/3(SW3_cmd) -> To File9/1, SW3_cmd/1
  [sw_conf] -> ROPOD 4SW/1(sw_conf)
  ROPOD 4SW/2(SW2_cmd) -> To File8/1, SW2_cmd/1
  sw_conf/1 -> Torque distribution using pseudoinverse/2(sw_conf), [sw_conf]
  [ropod_kin_param] -> wheel flip compensation/2(ropod_kin_param)
  Compare To Constant1/1 -> pivot damping cntr/2(disable)
  ddelta/1 -> pivot damping cntr/4(ddelta)
  [ropod_wheel_cntr_mode] -> Compare To Constant1/1
  platform_ddelta_cntr_param/1 -> pivot damping cntr/1(platform_ddelta_cntr_param)
  [ena_sw] -> pivot damping cntr/5(ena_w)
  Constant/1 -> pivot damping cntr/3(ddelta_ref)
  Torque distribution using pseudoinverse/1(varphi_tau_setp_out) -> Scope3/1, To File2/1, wheel flip compensation/1(varphi_tau_sp_in)
  [sw_conf] -> wheel flip compensation/4(sw_conf)
  [ena_sw] -> Own Constrainst Calculator/3(ena_sw)
  Divide/1 -> Own Constrainst Calculator/2(tau_max)
  Own Constrainst Calculator/1(enable_local_robot) -> enable_robot/1
  Own Constrainst Calculator/2(constraints_local_robot) -> constraints_robot/1
  [ropod_kin_param] -> Own Constrainst Calculator/1(ropod_kinmodel_param_vec)
  Inverse Kinematics 4SW/1(wheel_vel_sp) -> Selector1/1, wheel vel cntr/3(dvarphi_sp)
  [ropod_kin_param] -> Inverse Kinematics 4SW/1(param_in)
  wheel vel cntr/1(varphi_tau_setp_out) -> Selector/1, Scope2/1, To File4/1, [varphi_tau_dvarphi_cntr]
  platform_dvarphi_cntr_param/1 -> wheel vel cntr/1(platform_dxdy_cntr_param)
  dqr_sp_dvarphi_cntr/1 -> Scope/1, To File3/1, Inverse Kinematics 4SW/2(dqr_sp)
  dvarphi/1 -> Scope1/1, wheel vel cntr/5(dvarphi)
  [ena_sw] -> wheel vel cntr/4(ena_w)
  ropod_cntr_mode/1 -> [ropod_cntr_mode]
  [ropod_cntr_mode] -> Scope9/1, ROPOD 4SW/2(ropod_cntr_mode)
  [ropod_wheel_cntr_mode] -> Compare To Constant/1
  Compare To Constant/1 -> wheel vel cntr/2(disable)
  ropod_wheel_cntr_mode/1 -> [ropod_wheel_cntr_mode]
  [delta] -> Scope8/1, Inverse Kinematics 4SW/3(delta)
  [ropod_wheel_cntr_mode] -> Compare To Constant2/1
  Constant3/1 -> Switch1/1
  Constant1/1 -> Switch1/3
  Switch1/1 -> wheel flip compensation/3(flip_comp_factor)
  [ropod_wheel_cntr_mode] -> Multiport Switch/1
  Compare To Constant2/1 -> Switch1/2
  pivot damping cntr/1(varphi_tau_setp_out) -> [varphi_tau_ddelta_cntr]
  wheel flip compensation/1(varphi_tau_sp_out) -> Add/1
  Multiport Switch/1 -> Add/2
  Add/1 -> To File1/1, Scope10/1, ROPOD 4SW/3(varphi_tau_setp)
  Constant2/1 -> Multiport Switch/2
  [varphi_tau_ddelta_cntr] -> Multiport Switch/3
  [varphi_tau_dvarphi_cntr] -> Multiport Switch/4
  [varphi_tau_ddelta_cntr] -> Multiport Switch/5
  delta/1 -> Torque distribution using pseudoinverse/4(delta), [delta]
  Bus Selector1/1 -> Divide/1  "<max_current>"
  Bus Selector1/2 -> Divide/2  "<sw_tau_2_current>"
  [sw_conf] -> Bus Selector1/1
  Selector/1 -> Scope5/1
  Selector1/1 -> Scope7/1

== system ROPOD_Control_SIM/RopodVelocityController ==
  platform_dxdy_cntr_param : Inport
  platform_dtheta_cntr_param : Inport  Port=2
  base_conf : Inport  Port=3
  new_vel_cmd : Inport  Port=4
  vel_sp : Inport  Port=5
  initialize : Inport  Port=6
  ropod_enable : Inport  Port=7
  dqr_loc : Inport  Port=8
  Logical Operator : Logic  Operator=OR  AllPortsSameDT=off  OutDataTypeStr=boolean
  Logical Operator1 : Logic  Operator=NOT  AllPortsSameDT=off  OutDataTypeStr=boolean
  Platorm Velocity controller : Subsystem
  Subscriber vel commands1 : Subsystem
  w_platform_setp : Outport
  dqr_sp_dvarphi_cntr : Outport  Port=2
  wires:
  platform_dxdy_cntr_param/1 -> [platform_dxdy_cntr_param]
  platform_dtheta_cntr_param/1 -> [platform_dtheta_cntr_param]
  vel_sp/1 -> Subscriber vel commands1/3(dq_setp)
  base_conf/1 -> Subscriber vel commands1/1(base_conf)
  new_vel_cmd/1 -> Subscriber vel commands1/2(new_cmd)
  [platform_dxdy_cntr_param] -> Platorm Velocity controller/2(platform_dxdy_cntr_param)
  dqr_loc/1 -> Platorm Velocity controller/5(dqr_loc)
  Subscriber vel commands1/1(dq_loc_sp) -> dqr_sp_dvarphi_cntr/1, Platorm Velocity controller/4(dqr_sp)
  Platorm Velocity controller/1(w_platform_setp) -> w_platform_setp/1
  ropod_enable/1 -> Logical Operator1/1
  Logical Operator1/1 -> Logical Operator/2
  Logical Operator/1 -> Platorm Velocity controller/1(reset_int)
  initialize/1 -> Logical Operator/1
  [platform_dtheta_cntr_param] -> Platorm Velocity controller/3(platform_dtheta_cntr_param)

== system ROPOD_Control_SIM/Send_configuration_agent ==
  local_agent_configuration : Inport
  Enable : EnablePort
  UDP Send : dspnetwork/UDP Send  remoteURL='255.255.255.255'  remotePort=25002  localURL='0.0.0.0'  localPortSource=Automatically determine  localPort=-1  sampletime=-1  blockPlatform=[]  separateLengthPort=0
      settings: SourceProductName=DSP System Toolbox  SourceProductBaseCode=DS
  wires:
  local_agent_configuration/1 -> UDP Send/1

== system ROPOD_Control_SIM/Send_wrench_agents ==
  w_dq_agents_setp : Inport
  Enable : EnablePort
  UDP Send : dspnetwork/UDP Send  remoteURL='255.255.255.255'  remotePort=25001  localURL='0.0.0.0'  localPortSource=Automatically determine  localPort=-1  sampletime=-1  blockPlatform=[]  separateLengthPort=0
      settings: SourceProductName=DSP System Toolbox  SourceProductBaseCode=DS
  wires:
  w_dq_agents_setp/1 -> UDP Send/1

== system ROPOD_Control_SIM/Subsystem ==
  Ropod kinematic parameters : Subsystem
  Smart wheels conf1 : Subsystem
  ropod_kin_param : Outport
  sw_conf : Outport  Port=2
  wires:
  Ropod kinematic parameters/1(ropod_kin_param) -> ropod_kin_param/1
  Smart wheels conf1/1(sw_conf) -> sw_conf/1

== system ROPOD_Control_SIM/Subsystem1 ==
  In1 : Inport
  In2 : Inport  Port=2
  Compliant control : Subsystem
  Gain8 : Gain
      settings: OpenFcn=|
      | curvel = get_param(gcb,'Gain');
      | if strcmp(curvel,'1')
      | set_param(gcb,'Gain','0')
      | else
      | set_param(gcb,'Gain','1')
      | end
      | clear curvel
  Observer : Subsystem
  Out1 : Outport
  wires:
  In2/1 -> Compliant control/3(motion tuning bus)
  Observer/1(Force_obs) -> Compliant control/1(Forces)
  Compliant control/1(Force_out) -> Out1/1, Gain8/1
  Gain8/1 -> Observer/1(Input_force)
  In1/1 -> Compliant control/2(states), Observer/2(states)

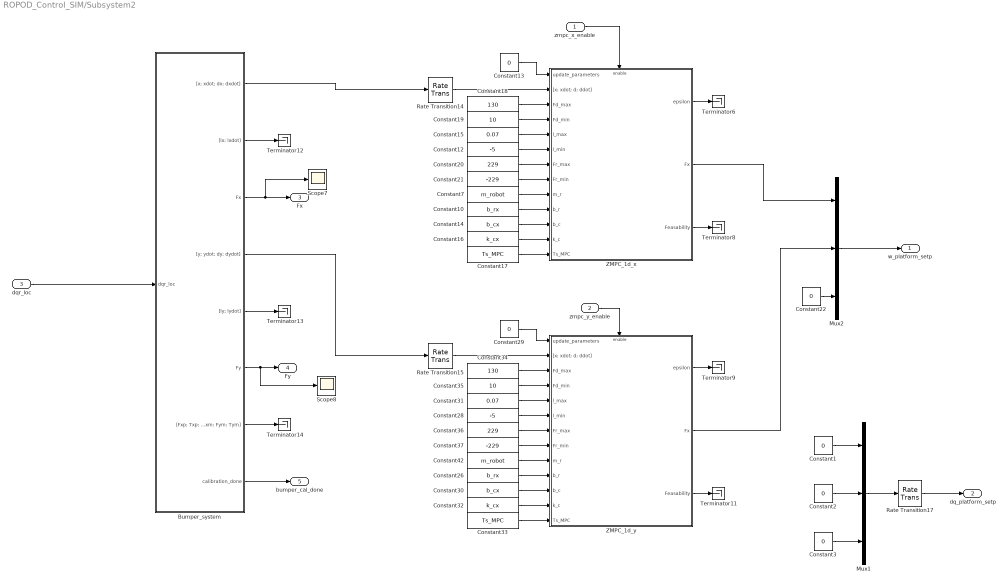
== system ROPOD_Control_SIM/Subsystem2 ==
  zmpc_x_enable : Inport
  zmpc_y_enable : Inport  Port=2
  dqr_loc : Inport  Port=3
  Bumper_system : Subsystem
  Constant{1..3,13,22,29} (6 alike) : Constant  Value=0
  Constant10 : Constant  Value=b_rx
  Constant12 : Constant  Value=-5
  Constant14 : Constant  Value=b_cx
  Constant15 : Constant  Value=0.07
  Constant16 : Constant  Value=k_cx
  Constant17 : Constant  Value=Ts_MPC
  Constant18 : Constant  Value=130
  Constant19 : Constant  Value=10
  Constant20 : Constant  Value=229
  Constant21 : Constant  Value=-229
  Constant26 : Constant  Value=b_rx
  Constant28 : Constant  Value=-5
  Constant30 : Constant  Value=b_cx
  Constant31 : Constant  Value=0.07
  Constant32 : Constant  Value=k_cx
  Constant33 : Constant  Value=Ts_MPC
  Constant34 : Constant  Value=130
  Constant35 : Constant  Value=10
  Constant36 : Constant  Value=229
  Constant37 : Constant  Value=-229
  Constant42 : Constant  Value=m_robot
  Constant7 : Constant  Value=m_robot
  Mux1 : Mux  Inputs=3
  Mux2 : Mux  Inputs=3
  Rate Transition14 : RateTransition
  Rate Transition15 : RateTransition
  Rate Transition17 : RateTransition  OutPortSampleTime=Tsflck
  Scope7 : Scope
  Scope8 : Scope
  Terminator{6,8..9,11..14} (7 alike) : Terminator
  ZMPC_1d_x : Subsystem  RTWFcnName=zone_mpc_1d_x  RTWFileName=zone_mpc_1d_x
      settings: RTWSystemCode=Nonreusable function  RTWFcnNameOpts=Use subsystem name  RTWFileNameOpts=Use subsystem name
  ZMPC_1d_y : Subsystem  RTWFcnName=zone_mpc_1d_x  RTWFileName=zone_mpc_1d_x
      settings: RTWSystemCode=Nonreusable function  RTWFcnNameOpts=Use subsystem name  RTWFileNameOpts=Use subsystem name
  w_platform_setp : Outport
  dq_platform_setp : Outport  Port=2
  Fx : Outport  Port=3
  Fy : Outport  Port=4
  bumper_cal_done : Outport  Port=5
  wires:
  Bumper_system/3(Fx) -> Scope7/1, Fx/1
  Bumper_system/5("[ly; lydot]") -> Terminator13/1
  Bumper_system/4("[y; ydot; dy; dydot]") -> Rate Transition15/1
  Constant28/1 -> ZMPC_1d_y/6(l_min)
  Constant26/1 -> ZMPC_1d_y/10(b_r)
  Constant30/1 -> ZMPC_1d_y/11(b_c)
  Constant31/1 -> ZMPC_1d_y/5(l_max)
  zmpc_y_enable/1 -> ZMPC_1d_y/Enable
  Mux2/1 -> w_platform_setp/1
  ZMPC_1d_y/3(Feasability) -> Terminator11/1
  Constant33/1 -> ZMPC_1d_y/13(Ts_MPC)
  Constant35/1 -> ZMPC_1d_y/4(Fd_min)
  Constant29/1 -> ZMPC_1d_y/1(update_parameters)
  Constant36/1 -> ZMPC_1d_y/7(Fr_max)
  Constant37/1 -> ZMPC_1d_y/8(Fr_min)
  Constant34/1 -> ZMPC_1d_y/3(Fd_max)
  Rate Transition15/1 -> ZMPC_1d_y/2("[x; xdot; d; ddot]")
  ZMPC_1d_y/1(epsilon) -> Terminator9/1
  Constant32/1 -> ZMPC_1d_y/12(k_c)
  Bumper_system/8(calibration_done) -> bumper_cal_done/1
  Bumper_system/7("[Fxp; Txp; Fyp Typ; Fxm; Txm; Fym; Tym] ") -> Terminator14/1
  dqr_loc/1 -> Bumper_system/1(dqr_loc)
  Constant19/1 -> ZMPC_1d_x/4(Fd_min)
  Constant21/1 -> ZMPC_1d_x/8(Fr_min)
  Constant20/1 -> ZMPC_1d_x/7(Fr_max)
  Bumper_system/1("[x; xdot; dx; dxdot]") -> Rate Transition14/1
  Constant14/1 -> ZMPC_1d_x/11(b_c)
  Constant16/1 -> ZMPC_1d_x/12(k_c)
  Constant42/1 -> ZMPC_1d_y/9(m_r)
  Rate Transition14/1 -> ZMPC_1d_x/2("[x; xdot; d; ddot]")
  Bumper_system/6(Fy) -> Fy/1, Scope8/1
  Constant7/1 -> ZMPC_1d_x/9(m_r)
  Constant10/1 -> ZMPC_1d_x/10(b_r)
  Constant17/1 -> ZMPC_1d_x/13(Ts_MPC)
  Constant15/1 -> ZMPC_1d_x/5(l_max)
  zmpc_x_enable/1 -> ZMPC_1d_x/Enable
  Bumper_system/2("[lx; lxdot]") -> Terminator12/1
  ZMPC_1d_x/1(epsilon) -> Terminator6/1
  Constant18/1 -> ZMPC_1d_x/3(Fd_max)
  Constant12/1 -> ZMPC_1d_x/6(l_min)
  Constant13/1 -> ZMPC_1d_x/1(update_parameters)
  ZMPC_1d_x/2(Fx) -> Mux2/1
  ZMPC_1d_x/3(Feasability) -> Terminator8/1
  ZMPC_1d_y/2(Fx) -> Mux2/2
  Constant22/1 -> Mux2/3
  Mux1/1 -> Rate Transition17/1
  Constant1/1 -> Mux1/1
  Constant2/1 -> Mux1/2
  Constant3/1 -> Mux1/3
  Rate Transition17/1 -> dq_platform_setp/1

== system ROPOD_Control_SIM/To_wrench_vel ==
  x : Inport
  y : Inport  Port=2
  theta : Inport  Port=3
  Gain : Gain  Gain=200
  Gain1 : Gain  Gain=200
  Gain2 : Gain  Gain=100
  Gain3 : Gain  Gain=0.2
  Gain4 : Gain  Gain=0.5
  Gain5 : Gain  Gain=0.5
  Gain6 : Gain
  Gain7 : Gain
  Mux : Mux  Inputs=3
  Mux1 : Mux  Inputs=3
  Mux3 : Mux  Inputs=2
  Rate Limiter : RateLimiter  RisingSlewLimit=200  FallingSlewLimit=-200  SampleTimeMode=inherited
  Rate Limiter1 : RateLimiter  SampleTimeMode=inherited
  Scope2 : Scope
  Out1 : Outport
  wires:
  Gain1/1 -> Mux/2
  Gain/1 -> Mux/1
  Gain2/1 -> Mux/3
  Gain3/1 -> Mux1/3
  Mux3/1 -> Out1/1
  Mux/1 -> Rate Limiter/1
  Mux1/1 -> Rate Limiter1/1
  y/1 -> Gain4/1, Gain1/1
  Gain5/1 -> Mux1/1
  Gain4/1 -> Mux1/2
  Rate Limiter/1 -> Scope2/1, Mux3/1
  Rate Limiter1/1 -> Mux3/2
  Gain6/1 -> Gain3/1, Gain2/1
  Gain7/1 -> Gain5/1, Gain/1
  x/1 -> Gain7/1
  theta/1 -> Gain6/1
